simulink model "snap_poco"  (R2013a)
settings: Solver=VariableStepDiscrete  SolverMode=SingleTasking  StartTime=0.0  StopTime=4096 * 16  RelTol=1e-3
undefined symbols (not defined in the file): pfb_coeff_gen_calc
libraries: xbsIndex_r4 x15564, xps_library x54, casper_library_misc x53, xbsReplacements_r4 x42, casper_library_delays x14, simulink x1
(part 31 of 142)

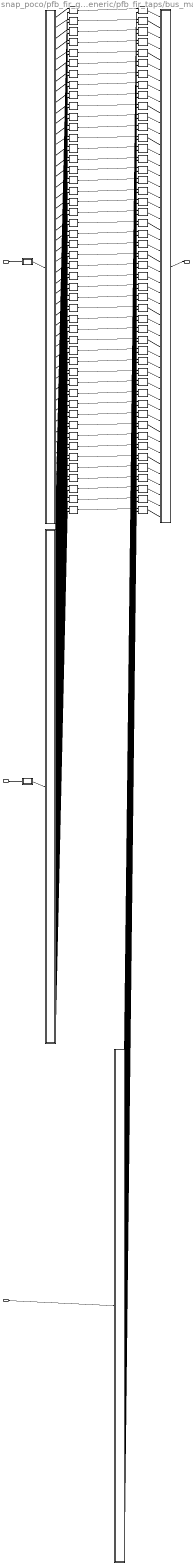
== system snap_poco/pfb_fir_generic/pfb_fir_taps/bus_madd ==
  a : Inport
  b : Inport  Port=2
  c : Inport  Port=3
  a*b+c_bussify : Subsystem  AncestorBlock=casper_library_flow_control/bus_create  mask(bus_create){inputNum=48}
      mask prompts: inputNum "Number of inputs:"
      mask init:
      | bus_create_init(gcb,...
      |     'inputNum', inputNum);
  a_debus : Subsystem  AncestorBlock=casper_library_flow_control/bus_expand  mask(bus_expand){mode=divisions of arbitrary size, outputNum=1, outputWidth=[8 8 8 8 8 8 8 8 8 8 8 8 8 8 8 8 8 8 8 8 8 8 8 8 8 8 8 8 8 8 8 8 8 8 8 8 8 8 8 8 8 8 8 8 8 8 8 8], outputBinaryPt=[7 7 7 7 7 7 7 7 7 7 7 7 7 7 7 7 7 7 7 7 7 7 7 7 7 7 7 7 7 7 7 7 7 7 7 7 7 7 7 7 7 7 7 7 7 7 7 7], outputArithmeticType=[1 1 1 1 1 1 1 1 1 1 1 1 1 1 1 1 1 1 1 1 1 1 1 1 1 1 1 1 1 1 1 1 1 1 1 1 1 1 1 1 1 1 1 1 1 1 1 1], show_format=on, outputToWorkspace=off, variablePrefix=, outputToModelAsWell=on}
      mask prompts: outputNum "Number of outputs:"; outputWidth "Output width [msb ... lsb]:"; outputBinaryPt "Output binary point position [msb ... lsb]:"; outputArithmeticType "Output arithmetic type (ufix=0, fix=1, bool=2) [msb ... lsb]:"; show_format "Print format string?"; outputToWorkspace "Output to workspace?"; variablePrefix "Variable name prefix:"; outputToModelAsWell "Output to model as well?"
      mask help:
      | Expands a 'bus' made using a bus_create or Xilinx
      | concat block.
      | The input will be divided into the specified number
      | of outputs with the specified arithmetic types.
      | Divisions are made from most significant bit.
      mask init: same as snap_poco/fft_biplex_real_2x/even_pol_debus
      settings: AttributesFormatString=48 outputs: f8.7,f8.7,f8.7,f8.7,f8.7,f8.7,f8.7,f8.7,f8.7,f8.7,f8.7,f8.7,f8.7,f8.7,f8.7,f8.7,f8.7,f8.7,f8.7,f8.7,f8.7,f8.7,f8.7,f8.7,f8.7,f8.7,f8.7,f8.7,f8.7,f8.7,f8.7,f8.7,f8.7,f8.7,f8.7,f8.7,f8.7,f8.7,f8.7,f8.7,f8.7,f8.7,f8.7,f8.7,f8.7,f8.7,f8.7,f8.7,
      mask TypeOptions mode: divisions of equal size | divisions of arbitrary size
      mask Callback mode: bus_expand_callback();
      mask Callback outputWidth: bus_expand_callback();
      mask Callback outputToWorkspace: bus_expand_callback();
  addsub{1..12} (12 alike) : xbsIndex_r4/AddSub  mode=Addition  use_carryin=off  use_carryout=off  en=off  latency=2  precision=User Defined  arith_type="Signed  (2's comp)"  n_bits=26  bin_pt=24  quantization=Truncate  overflow=Wrap  use_behavioral_HDL=on  hw_selection=Fabric  pipelined=on  dbl_ovrd=off  block_type=addsub
  addsub{13..24} (12 alike) : xbsIndex_r4/AddSub  mode=Addition  use_carryin=off  use_carryout=off  en=off  latency=2  precision=User Defined  arith_type="Signed  (2's comp)"  n_bits=27  bin_pt=24  quantization=Truncate  overflow=Wrap  use_behavioral_HDL=on  hw_selection=Fabric  pipelined=on  dbl_ovrd=off  block_type=addsub
  addsub{25..36} (12 alike) : xbsIndex_r4/AddSub  mode=Addition  use_carryin=off  use_carryout=off  en=off  latency=2  precision=User Defined  arith_type="Signed  (2's comp)"  n_bits=28  bin_pt=24  quantization=Truncate  overflow=Wrap  use_behavioral_HDL=on  hw_selection=Fabric  pipelined=on  dbl_ovrd=off  block_type=addsub
  addsub{37..48} (12 alike) : xbsIndex_r4/AddSub  mode=Addition  use_carryin=off  use_carryout=off  en=off  latency=2  precision=User Defined  arith_type="Signed  (2's comp)"  n_bits=29  bin_pt=24  quantization=Truncate  overflow=Wrap  use_behavioral_HDL=on  hw_selection=Fabric  pipelined=on  dbl_ovrd=off  block_type=addsub
  b_debus : Subsystem  AncestorBlock=casper_library_flow_control/bus_expand  mask(bus_expand){mode=divisions of arbitrary size, outputNum=1, outputWidth=[18 18 18 18 18 18 18 18 18 18 18 18 18 18 18 18 18 18 18 18 18 18 18 18 18 18 18 18 18 18 18 18 18 18 18 18 18 18 18 18 18 18 18 18 18 18 18 18], outputBinaryPt=[17 17 17 17 17 17 17 17 17 17 17 17 17 17 17 17 17 17 17 17 17 17 17 17 17 17 17 17 17 17 17 17 17 17 17 17 17 17 17 17 17 17 17 17 17 17 17 17], outputArithmeticType=[1 1 1 1 1 1 1 1 1 1 1 1 1 1 1 1 1 1 1 1 1 1 1 1 1 1 1 1 1 1 1 1 1 1 1 1 1 1 1 1 1 1 1 1 1 1 1 1], show_format=on, outputToWorkspace=off, variablePrefix=, outputToModelAsWell=on}
      mask prompts: outputNum "Number of outputs:"; outputWidth "Output width [msb ... lsb]:"; outputBinaryPt "Output binary point position [msb ... lsb]:"; outputArithmeticType "Output arithmetic type (ufix=0, fix=1, bool=2) [msb ... lsb]:"; show_format "Print format string?"; outputToWorkspace "Output to workspace?"; variablePrefix "Variable name prefix:"; outputToModelAsWell "Output to model as well?"
      mask help:
      | Expands a 'bus' made using a bus_create or Xilinx
      | concat block.
      | The input will be divided into the specified number
      | of outputs with the specified arithmetic types.
      | Divisions are made from most significant bit.
      mask init: same as snap_poco/fft_biplex_real_2x/even_pol_debus
      settings: AttributesFormatString=48 outputs: f18.17,f18.17,f18.17,f18.17,f18.17,f18.17,f18.17,f18.17,f18.17,f18.17,f18.17,f18.17,f18.17,f18.17,f18.17,f18.17,f18.17,f18.17,f18.17,f18.17,f18.17,f18.17,f18.17,f18.17,f18.17,f18.17,f18.17,f18.17,f18.17,f18.17,f18.17,f18.17,f18.17,f18.17,f18.17,f18.17,f18.17,f18.17,f18.17,f18.17,f18.17,f18.17,f18.17,f18.17,f18.17,f18.17,f18.17,f18.17,
      mask TypeOptions mode: divisions of equal size | divisions of arbitrary size
      mask Callback mode: bus_expand_callback();
      mask Callback outputWidth: bus_expand_callback();
      mask Callback outputToWorkspace: bus_expand_callback();
  c_debus : Subsystem  AncestorBlock=casper_library_flow_control/bus_expand  mask(bus_expand){mode=divisions of arbitrary size, outputNum=1, outputWidth=[26 26 26 26 26 26 26 26 26 26 26 26 26 26 26 26 26 26 26 26 26 26 26 26 27 27 27 27 27 27 27 27 27 27 27 27 28 28 28 28 28 28 28 28 28 28 28 28], outputBinaryPt=[24 24 24 24 24 24 24 24 24 24 24 24 24 24 24 24 24 24 24 24 24 24 24 24 24 24 24 24 24 24 24 24 24 24 24 24 24 24 24 24 24 24 24 24 24 24 24 24], outputArithmeticType=[1 1 1 1 1 1 1 1 1 1 1 1 1 1 1 1 1 1 1 1 1 1 1 1 1 1 1 1 1 1 1 1 1 1 1 1 1 1 1 1 1 1 1 1 1 1 1 1], show_format=on, outputToWorkspace=off, variablePrefix=, outputToModelAsWell=on}
      mask prompts: outputNum "Number of outputs:"; outputWidth "Output width [msb ... lsb]:"; outputBinaryPt "Output binary point position [msb ... lsb]:"; outputArithmeticType "Output arithmetic type (ufix=0, fix=1, bool=2) [msb ... lsb]:"; show_format "Print format string?"; outputToWorkspace "Output to workspace?"; variablePrefix "Variable name prefix:"; outputToModelAsWell "Output to model as well?"
      mask help:
      | Expands a 'bus' made using a bus_create or Xilinx
      | concat block.
      | The input will be divided into the specified number
      | of outputs with the specified arithmetic types.
      | Divisions are made from most significant bit.
      mask init: same as snap_poco/fft_biplex_real_2x/even_pol_debus
      settings: AttributesFormatString=48 outputs: f26.24,f26.24,f26.24,f26.24,f26.24,f26.24,f26.24,f26.24,f26.24,f26.24,f26.24,f26.24,f26.24,f26.24,f26.24,f26.24,f26.24,f26.24,f26.24,f26.24,f26.24,f26.24,f26.24,f26.24,f27.24,f27.24,f27.24,f27.24,f27.24,f27.24,f27.24,f27.24,f27.24,f27.24,f27.24,f27.24,f28.24,f28.24,f28.24,f28.24,f28.24,f28.24,f28.24,f28.24,f28.24,f28.24,f28.24,f28.24,
      mask TypeOptions mode: divisions of equal size | divisions of arbitrary size
      mask Callback mode: bus_expand_callback();
      mask Callback outputWidth: bus_expand_callback();
      mask Callback outputToWorkspace: bus_expand_callback();
  mult{1..48} (48 alike) : xbsIndex_r4/Mult  precision=Full  arith_type="Signed  (2's comp)"  n_bits=16  bin_pt=14  quantization=Truncate  overflow=Wrap  en=off  latency=3  use_behavioral_HDL=on  opt=Speed  use_embedded=off  optimum_pipeline=off  pipeline=on  dbl_ovrd=off  use_rpm=on  placement_style=Triangular  block_type=mult
  repa : Subsystem  AncestorBlock=casper_library_bus/bus_replicate  mask(bus_replicate){replication=1, latency=1, misc=off, implementation=core}
      mask prompts: replication "replication factor"; misc "misc support"; implementation "delay implementation"
      mask help: Output bus formed by replicating input bus a number of times
      mask init:
      | bus_replicate_init(gcb, ...
      |     'replication', replication, ...
      |     'latency', latency, ...
      |     'implementation', implementation, ...
      |     'misc', misc);
      mask TypeOptions implementation: core | behavioral
  repb : Subsystem  AncestorBlock=casper_library_bus/bus_replicate  mask(bus_replicate){replication=1, latency=1, misc=off, implementation=core}
      mask prompts: replication "replication factor"; misc "misc support"; implementation "delay implementation"
      mask help: Output bus formed by replicating input bus a number of times
      mask init:
      | bus_replicate_init(gcb, ...
      |     'replication', replication, ...
      |     'latency', latency, ...
      |     'implementation', implementation, ...
      |     'misc', misc);
      mask TypeOptions implementation: core | behavioral
  a*b+c : Outport
  wires:
  a/1 -> repa/1(in)
  b/1 -> repb/1(in)
  repa/1(out) -> a_debus/1(bus_in)
  repb/1(out) -> b_debus/1(bus_in)
  a_debus/1(msb_out48) -> mult1/1
  b_debus/1(msb_out48) -> mult1/2
  a_debus/2(out47) -> mult2/1
  b_debus/2(out47) -> mult2/2
  a_debus/3(out46) -> mult3/1
  b_debus/3(out46) -> mult3/2
  a_debus/4(out45) -> mult4/1
  b_debus/4(out45) -> mult4/2
  a_debus/5(out44) -> mult5/1
  b_debus/5(out44) -> mult5/2
  a_debus/6(out43) -> mult6/1
  b_debus/6(out43) -> mult6/2
  a_debus/7(out42) -> mult7/1
  b_debus/7(out42) -> mult7/2
  a_debus/8(out41) -> mult8/1
  b_debus/8(out41) -> mult8/2
  a_debus/9(out40) -> mult9/1
  b_debus/9(out40) -> mult9/2
  a_debus/10(out39) -> mult10/1
  b_debus/10(out39) -> mult10/2
  a_debus/11(out38) -> mult11/1
  b_debus/11(out38) -> mult11/2
  a_debus/12(out37) -> mult12/1
  b_debus/12(out37) -> mult12/2
  a_debus/13(out36) -> mult13/1
  b_debus/13(out36) -> mult13/2
  a_debus/14(out35) -> mult14/1
  b_debus/14(out35) -> mult14/2
  a_debus/15(out34) -> mult15/1
  b_debus/15(out34) -> mult15/2
  a_debus/16(out33) -> mult16/1
  b_debus/16(out33) -> mult16/2
  a_debus/17(out32) -> mult17/1
  b_debus/17(out32) -> mult17/2
  a_debus/18(out31) -> mult18/1
  b_debus/18(out31) -> mult18/2
  a_debus/19(out30) -> mult19/1
  b_debus/19(out30) -> mult19/2
  a_debus/20(out29) -> mult20/1
  b_debus/20(out29) -> mult20/2
  a_debus/21(out28) -> mult21/1
  b_debus/21(out28) -> mult21/2
  a_debus/22(out27) -> mult22/1
  b_debus/22(out27) -> mult22/2
  a_debus/23(out26) -> mult23/1
  b_debus/23(out26) -> mult23/2
  a_debus/24(out25) -> mult24/1
  b_debus/24(out25) -> mult24/2
  a_debus/25(out24) -> mult25/1
  b_debus/25(out24) -> mult25/2
  a_debus/26(out23) -> mult26/1
  b_debus/26(out23) -> mult26/2
  a_debus/27(out22) -> mult27/1
  b_debus/27(out22) -> mult27/2
  a_debus/28(out21) -> mult28/1
  b_debus/28(out21) -> mult28/2
  a_debus/29(out20) -> mult29/1
  b_debus/29(out20) -> mult29/2
  a_debus/30(out19) -> mult30/1
  b_debus/30(out19) -> mult30/2
  a_debus/31(out18) -> mult31/1
  b_debus/31(out18) -> mult31/2
  a_debus/32(out17) -> mult32/1
  b_debus/32(out17) -> mult32/2
  a_debus/33(out16) -> mult33/1
  b_debus/33(out16) -> mult33/2
  a_debus/34(out15) -> mult34/1
  b_debus/34(out15) -> mult34/2
  a_debus/35(out14) -> mult35/1
  b_debus/35(out14) -> mult35/2
  a_debus/36(out13) -> mult36/1
  b_debus/36(out13) -> mult36/2
  a_debus/37(out12) -> mult37/1
  b_debus/37(out12) -> mult37/2
  a_debus/38(out11) -> mult38/1
  b_debus/38(out11) -> mult38/2
  a_debus/39(out10) -> mult39/1
  b_debus/39(out10) -> mult39/2
  a_debus/40(out9) -> mult40/1
  b_debus/40(out9) -> mult40/2
  a_debus/41(out8) -> mult41/1
  b_debus/41(out8) -> mult41/2
  a_debus/42(out7) -> mult42/1
  b_debus/42(out7) -> mult42/2
  a_debus/43(out6) -> mult43/1
  b_debus/43(out6) -> mult43/2
  a_debus/44(out5) -> mult44/1
  b_debus/44(out5) -> mult44/2
  a_debus/45(out4) -> mult45/1
  b_debus/45(out4) -> mult45/2
  a_debus/46(out3) -> mult46/1
  b_debus/46(out3) -> mult46/2
  a_debus/47(out2) -> mult47/1
  b_debus/47(out2) -> mult47/2
  a_debus/48(lsb_out1) -> mult48/1
  b_debus/48(lsb_out1) -> mult48/2
  c/1 -> c_debus/1(bus_in)
  mult1/1 -> addsub1/1
  c_debus/1(msb_out48) -> addsub1/2
  mult2/1 -> addsub2/1
  c_debus/2(out47) -> addsub2/2
  mult3/1 -> addsub3/1
  c_debus/3(out46) -> addsub3/2
  mult4/1 -> addsub4/1
  c_debus/4(out45) -> addsub4/2
  mult5/1 -> addsub5/1
  c_debus/5(out44) -> addsub5/2
  mult6/1 -> addsub6/1
  c_debus/6(out43) -> addsub6/2
  mult7/1 -> addsub7/1
  c_debus/7(out42) -> addsub7/2
  mult8/1 -> addsub8/1
  c_debus/8(out41) -> addsub8/2
  mult9/1 -> addsub9/1
  c_debus/9(out40) -> addsub9/2
  mult10/1 -> addsub10/1
  c_debus/10(out39) -> addsub10/2
  mult11/1 -> addsub11/1
  c_debus/11(out38) -> addsub11/2
  mult12/1 -> addsub12/1
  c_debus/12(out37) -> addsub12/2
  mult13/1 -> addsub13/1
  c_debus/13(out36) -> addsub13/2
  mult14/1 -> addsub14/1
  c_debus/14(out35) -> addsub14/2
  mult15/1 -> addsub15/1
  c_debus/15(out34) -> addsub15/2
  mult16/1 -> addsub16/1
  c_debus/16(out33) -> addsub16/2
  mult17/1 -> addsub17/1
  c_debus/17(out32) -> addsub17/2
  mult18/1 -> addsub18/1
  c_debus/18(out31) -> addsub18/2
  mult19/1 -> addsub19/1
  c_debus/19(out30) -> addsub19/2
  mult20/1 -> addsub20/1
  c_debus/20(out29) -> addsub20/2
  mult21/1 -> addsub21/1
  c_debus/21(out28) -> addsub21/2
  mult22/1 -> addsub22/1
  c_debus/22(out27) -> addsub22/2
  mult23/1 -> addsub23/1
  c_debus/23(out26) -> addsub23/2
  mult24/1 -> addsub24/1
  c_debus/24(out25) -> addsub24/2
  mult25/1 -> addsub25/1
  c_debus/25(out24) -> addsub25/2
  mult26/1 -> addsub26/1
  c_debus/26(out23) -> addsub26/2
  mult27/1 -> addsub27/1
  c_debus/27(out22) -> addsub27/2
  mult28/1 -> addsub28/1
  c_debus/28(out21) -> addsub28/2
  mult29/1 -> addsub29/1
  c_debus/29(out20) -> addsub29/2
  mult30/1 -> addsub30/1
  c_debus/30(out19) -> addsub30/2
  mult31/1 -> addsub31/1
  c_debus/31(out18) -> addsub31/2
  mult32/1 -> addsub32/1
  c_debus/32(out17) -> addsub32/2
  mult33/1 -> addsub33/1
  c_debus/33(out16) -> addsub33/2
  mult34/1 -> addsub34/1
  c_debus/34(out15) -> addsub34/2
  mult35/1 -> addsub35/1
  c_debus/35(out14) -> addsub35/2
  mult36/1 -> addsub36/1
  c_debus/36(out13) -> addsub36/2
  mult37/1 -> addsub37/1
  c_debus/37(out12) -> addsub37/2
  mult38/1 -> addsub38/1
  c_debus/38(out11) -> addsub38/2
  mult39/1 -> addsub39/1
  c_debus/39(out10) -> addsub39/2
  mult40/1 -> addsub40/1
  c_debus/40(out9) -> addsub40/2
  mult41/1 -> addsub41/1
  c_debus/41(out8) -> addsub41/2
  mult42/1 -> addsub42/1
  c_debus/42(out7) -> addsub42/2
  mult43/1 -> addsub43/1
  c_debus/43(out6) -> addsub43/2
  mult44/1 -> addsub44/1
  c_debus/44(out5) -> addsub44/2
  mult45/1 -> addsub45/1
  c_debus/45(out4) -> addsub45/2
  mult46/1 -> addsub46/1
  c_debus/46(out3) -> addsub46/2
  mult47/1 -> addsub47/1
  c_debus/47(out2) -> addsub47/2
  mult48/1 -> addsub48/1
  c_debus/48(lsb_out1) -> addsub48/2
  addsub1/1 -> a*b+c_bussify/1(in1)
  addsub2/1 -> a*b+c_bussify/2(in2)
  addsub3/1 -> a*b+c_bussify/3(in3)
  addsub4/1 -> a*b+c_bussify/4(in4)
  addsub5/1 -> a*b+c_bussify/5(in5)
  addsub6/1 -> a*b+c_bussify/6(in6)
  addsub7/1 -> a*b+c_bussify/7(in7)
  addsub8/1 -> a*b+c_bussify/8(in8)
  addsub9/1 -> a*b+c_bussify/9(in9)
  addsub10/1 -> a*b+c_bussify/10(in10)
  addsub11/1 -> a*b+c_bussify/11(in11)
  addsub12/1 -> a*b+c_bussify/12(in12)
  addsub13/1 -> a*b+c_bussify/13(in13)
  addsub14/1 -> a*b+c_bussify/14(in14)
  addsub15/1 -> a*b+c_bussify/15(in15)
  addsub16/1 -> a*b+c_bussify/16(in16)
  addsub17/1 -> a*b+c_bussify/17(in17)
  addsub18/1 -> a*b+c_bussify/18(in18)
  addsub19/1 -> a*b+c_bussify/19(in19)
  addsub20/1 -> a*b+c_bussify/20(in20)
  addsub21/1 -> a*b+c_bussify/21(in21)
  addsub22/1 -> a*b+c_bussify/22(in22)
  addsub23/1 -> a*b+c_bussify/23(in23)
  addsub24/1 -> a*b+c_bussify/24(in24)
  addsub25/1 -> a*b+c_bussify/25(in25)
  addsub26/1 -> a*b+c_bussify/26(in26)
  addsub27/1 -> a*b+c_bussify/27(in27)
  addsub28/1 -> a*b+c_bussify/28(in28)
  addsub29/1 -> a*b+c_bussify/29(in29)
  addsub30/1 -> a*b+c_bussify/30(in30)
  addsub31/1 -> a*b+c_bussify/31(in31)
  addsub32/1 -> a*b+c_bussify/32(in32)
  addsub33/1 -> a*b+c_bussify/33(in33)
  addsub34/1 -> a*b+c_bussify/34(in34)
  addsub35/1 -> a*b+c_bussify/35(in35)
  addsub36/1 -> a*b+c_bussify/36(in36)
  addsub37/1 -> a*b+c_bussify/37(in37)
  addsub38/1 -> a*b+c_bussify/38(in38)
  addsub39/1 -> a*b+c_bussify/39(in39)
  addsub40/1 -> a*b+c_bussify/40(in40)
  addsub41/1 -> a*b+c_bussify/41(in41)
  addsub42/1 -> a*b+c_bussify/42(in42)
  addsub43/1 -> a*b+c_bussify/43(in43)
  addsub44/1 -> a*b+c_bussify/44(in44)
  addsub45/1 -> a*b+c_bussify/45(in45)
  addsub46/1 -> a*b+c_bussify/46(in46)
  addsub47/1 -> a*b+c_bussify/47(in47)
  addsub48/1 -> a*b+c_bussify/48(in48)
  a*b+c_bussify/1(bus_out) -> a*b+c/1

== system snap_poco/pfb_fir_generic/pfb_fir_taps/ddata0 ==
  din : Inport
  del{1..24} (24 alike) : xbsIndex_r4/Delay  rst=off  infoeditControl=Selection of Reset will increase slice count due to use of real FFs and instead of SRLs  en=off  latency=2  reg_retiming=on  dbl_ovrd=off  block_type=delay
  din_expand : Subsystem  AncestorBlock=casper_library_flow_control/bus_expand  mask(bus_expand){mode=divisions of arbitrary size, outputNum=1, outputWidth=[8  8  8  8  8  8  8  8  8  8  8  8  8  8  8  8  8  8  8  8  8  8  8  8], outputBinaryPt=[0  0  0  0  0  0  0  0  0  0  0  0  0  0  0  0  0  0  0  0  0  0  0  0], outputArithmeticType=[0  0  0  0  0  0  0  0  0  0  0  0  0  0  0  0  0  0  0  0  0  0  0  0], show_format=on, outputToWorkspace=off, variablePrefix=, outputToModelAsWell=on}
      mask prompts: outputNum "Number of outputs:"; outputWidth "Output width [msb ... lsb]:"; outputBinaryPt "Output binary point position [msb ... lsb]:"; outputArithmeticType "Output arithmetic type (ufix=0, fix=1, bool=2) [msb ... lsb]:"; show_format "Print format string?"; outputToWorkspace "Output to workspace?"; variablePrefix "Variable name prefix:"; outputToModelAsWell "Output to model as well?"
      mask help:
      | Expands a 'bus' made using a bus_create or Xilinx
      | concat block.
      | The input will be divided into the specified number
      | of outputs with the specified arithmetic types.
      | Divisions are made from most significant bit.
      mask init: same as snap_poco/fft_biplex_real_2x/even_pol_debus
      settings: AttributesFormatString=24 outputs: uf8.0,uf8.0,uf8.0,uf8.0,uf8.0,uf8.0,uf8.0,uf8.0,uf8.0,uf8.0,uf8.0,uf8.0,uf8.0,uf8.0,uf8.0,uf8.0,uf8.0,uf8.0,uf8.0,uf8.0,uf8.0,uf8.0,uf8.0,uf8.0,
      mask TypeOptions mode: divisions of equal size | divisions of arbitrary size
      mask Callback mode: bus_expand_callback();
      mask Callback outputWidth: bus_expand_callback();
      mask Callback outputToWorkspace: bus_expand_callback();
  dout_compress : Subsystem  AncestorBlock=casper_library_flow_control/bus_create  mask(bus_create){inputNum=24}
      mask prompts: inputNum "Number of inputs:"
      mask init:
      | bus_create_init(gcb,...
      |     'inputNum', inputNum);
  dout : Outport
  wires:
  din/1 -> din_expand/1(bus_in)
  din_expand/1(msb_out24) -> del1/1
  din_expand/2(out23) -> del2/1
  din_expand/3(out22) -> del3/1
  din_expand/4(out21) -> del4/1
  din_expand/5(out20) -> del5/1
  din_expand/6(out19) -> del6/1
  din_expand/7(out18) -> del7/1
  din_expand/8(out17) -> del8/1
  din_expand/9(out16) -> del9/1
  din_expand/10(out15) -> del10/1
  din_expand/11(out14) -> del11/1
  din_expand/12(out13) -> del12/1
  din_expand/13(out12) -> del13/1
  din_expand/14(out11) -> del14/1
  din_expand/15(out10) -> del15/1
  din_expand/16(out9) -> del16/1
  din_expand/17(out8) -> del17/1
  din_expand/18(out7) -> del18/1
  din_expand/19(out6) -> del19/1
  din_expand/20(out5) -> del20/1
  din_expand/21(out4) -> del21/1
  din_expand/22(out3) -> del22/1
  din_expand/23(out2) -> del23/1
  din_expand/24(lsb_out1) -> del24/1
  del1/1 -> dout_compress/1(in1)
  del2/1 -> dout_compress/2(in2)
  del3/1 -> dout_compress/3(in3)
  del4/1 -> dout_compress/4(in4)
  del5/1 -> dout_compress/5(in5)
  del6/1 -> dout_compress/6(in6)
  del7/1 -> dout_compress/7(in7)
  del8/1 -> dout_compress/8(in8)
  del9/1 -> dout_compress/9(in9)
  del10/1 -> dout_compress/10(in10)
  del11/1 -> dout_compress/11(in11)
  del12/1 -> dout_compress/12(in12)
  del13/1 -> dout_compress/13(in13)
  del14/1 -> dout_compress/14(in14)
  del15/1 -> dout_compress/15(in15)
  del16/1 -> dout_compress/16(in16)
  del17/1 -> dout_compress/17(in17)
  del18/1 -> dout_compress/18(in18)
  del19/1 -> dout_compress/19(in19)
  del20/1 -> dout_compress/20(in20)
  del21/1 -> dout_compress/21(in21)
  del22/1 -> dout_compress/22(in22)
  del23/1 -> dout_compress/23(in23)
  del24/1 -> dout_compress/24(in24)
  dout_compress/1(bus_out) -> dout/1

== system snap_poco/pfb_fir_generic/pfb_fir_taps/ddata1 ==
  din : Inport
  del{1..36} (36 alike) : xbsIndex_r4/Delay  rst=off  infoeditControl=Selection of Reset will increase slice count due to use of real FFs and instead of SRLs  en=off  latency=2  reg_retiming=on  dbl_ovrd=off  block_type=delay
  din_expand : Subsystem  AncestorBlock=casper_library_flow_control/bus_expand  mask(bus_expand){mode=divisions of arbitrary size, outputNum=1, outputWidth=[8  8  8  8  8  8  8  8  8  8  8  8  8  8  8  8  8  8  8  8  8  8  8  8  8  8  8  8  8  8  8  8  8  8  8  8], outputBinaryPt=[0  0  0  0  0  0  0  0  0  0  0  0  0  0  0  0  0  0  0  0  0  0  0  0  0  0  0  0  0  0  0  0  0  0  0  0], outputArithmeticType=[0  0  0  0  0  0  0  0  0  0  0  0  0  0  0  0  0  0  0  0  0  0  0  0  0  0  0  0  0  0  0  0  0  0  0  0], show_format=on, outputToWorkspace=off, variablePrefix=, outputToModelAsWell=on}
      mask prompts: outputNum "Number of outputs:"; outputWidth "Output width [msb ... lsb]:"; outputBinaryPt "Output binary point position [msb ... lsb]:"; outputArithmeticType "Output arithmetic type (ufix=0, fix=1, bool=2) [msb ... lsb]:"; show_format "Print format string?"; outputToWorkspace "Output to workspace?"; variablePrefix "Variable name prefix:"; outputToModelAsWell "Output to model as well?"
      mask help:
      | Expands a 'bus' made using a bus_create or Xilinx
      | concat block.
      | The input will be divided into the specified number
      | of outputs with the specified arithmetic types.
      | Divisions are made from most significant bit.
      mask init: same as snap_poco/fft_biplex_real_2x/even_pol_debus
      settings: AttributesFormatString=36 outputs: uf8.0,uf8.0,uf8.0,uf8.0,uf8.0,uf8.0,uf8.0,uf8.0,uf8.0,uf8.0,uf8.0,uf8.0,uf8.0,uf8.0,uf8.0,uf8.0,uf8.0,uf8.0,uf8.0,uf8.0,uf8.0,uf8.0,uf8.0,uf8.0,uf8.0,uf8.0,uf8.0,uf8.0,uf8.0,uf8.0,uf8.0,uf8.0,uf8.0,uf8.0,uf8.0,uf8.0,
      mask TypeOptions mode: divisions of equal size | divisions of arbitrary size
      mask Callback mode: bus_expand_callback();
      mask Callback outputWidth: bus_expand_callback();
      mask Callback outputToWorkspace: bus_expand_callback();
  dout_compress : Subsystem  AncestorBlock=casper_library_flow_control/bus_create  mask(bus_create){inputNum=36}
      mask prompts: inputNum "Number of inputs:"
      mask init:
      | bus_create_init(gcb,...
      |     'inputNum', inputNum);
  dout : Outport
  wires:
  din/1 -> din_expand/1(bus_in)
  din_expand/1(msb_out36) -> del1/1
  din_expand/2(out35) -> del2/1
  din_expand/3(out34) -> del3/1
  din_expand/4(out33) -> del4/1
  din_expand/5(out32) -> del5/1
  din_expand/6(out31) -> del6/1
  din_expand/7(out30) -> del7/1
  din_expand/8(out29) -> del8/1
  din_expand/9(out28) -> del9/1
  din_expand/10(out27) -> del10/1
  din_expand/11(out26) -> del11/1
  din_expand/12(out25) -> del12/1
  din_expand/13(out24) -> del13/1
  din_expand/14(out23) -> del14/1
  din_expand/15(out22) -> del15/1
  din_expand/16(out21) -> del16/1
  din_expand/17(out20) -> del17/1
  din_expand/18(out19) -> del18/1
  din_expand/19(out18) -> del19/1
  din_expand/20(out17) -> del20/1
  din_expand/21(out16) -> del21/1
  din_expand/22(out15) -> del22/1
  din_expand/23(out14) -> del23/1
  din_expand/24(out13) -> del24/1
  din_expand/25(out12) -> del25/1
  din_expand/26(out11) -> del26/1
  din_expand/27(out10) -> del27/1
  din_expand/28(out9) -> del28/1
  din_expand/29(out8) -> del29/1
  din_expand/30(out7) -> del30/1
  din_expand/31(out6) -> del31/1
  din_expand/32(out5) -> del32/1
  din_expand/33(out4) -> del33/1
  din_expand/34(out3) -> del34/1
  din_expand/35(out2) -> del35/1
  din_expand/36(lsb_out1) -> del36/1
  del1/1 -> dout_compress/1(in1)
  del2/1 -> dout_compress/2(in2)
  del3/1 -> dout_compress/3(in3)
  del4/1 -> dout_compress/4(in4)
  del5/1 -> dout_compress/5(in5)
  del6/1 -> dout_compress/6(in6)
  del7/1 -> dout_compress/7(in7)
  del8/1 -> dout_compress/8(in8)
  del9/1 -> dout_compress/9(in9)
  del10/1 -> dout_compress/10(in10)
  del11/1 -> dout_compress/11(in11)
  del12/1 -> dout_compress/12(in12)
  del13/1 -> dout_compress/13(in13)
  del14/1 -> dout_compress/14(in14)
  del15/1 -> dout_compress/15(in15)
  del16/1 -> dout_compress/16(in16)
  del17/1 -> dout_compress/17(in17)
  del18/1 -> dout_compress/18(in18)
  del19/1 -> dout_compress/19(in19)
  del20/1 -> dout_compress/20(in20)
  del21/1 -> dout_compress/21(in21)
  del22/1 -> dout_compress/22(in22)
  del23/1 -> dout_compress/23(in23)
  del24/1 -> dout_compress/24(in24)
  del25/1 -> dout_compress/25(in25)
  del26/1 -> dout_compress/26(in26)
  del27/1 -> dout_compress/27(in27)
  del28/1 -> dout_compress/28(in28)
  del29/1 -> dout_compress/29(in29)
  del30/1 -> dout_compress/30(in30)
  del31/1 -> dout_compress/31(in31)
  del32/1 -> dout_compress/32(in32)
  del33/1 -> dout_compress/33(in33)
  del34/1 -> dout_compress/34(in34)
  del35/1 -> dout_compress/35(in35)
  del36/1 -> dout_compress/36(in36)
  dout_compress/1(bus_out) -> dout/1

== system snap_poco/pfb_fir_generic/pfb_fir_taps/delay_bram ==
  addr : Inport
  din : Inport  Port=2
  we : Inport  Port=3
  bram{0..31} (32 alike) : xbsIndex_r4/Single Port RAM  depth=2048  initVector=getfield(get_param(gcb, 'UserData'), 'initVector')  distributed_mem=Block RAM  write_mode=Read Before Write  rst=off  init_reg=0  en=off  latency=1  optimize=Area  dbl_ovrd=off  block_type=spram
  ddin : xbsIndex_r4/Delay  rst=off  infoeditControl=Selection of Reset will increase slice count due to use of real FFs and instead of SRLs  en=off  latency=0  reg_retiming=on  dbl_ovrd=off  block_type=delay
  debus_addr : Subsystem  AncestorBlock=casper_library_flow_control/bus_expand  mask(bus_expand){mode=divisions of equal size, outputNum=32, outputWidth=[11 11 11 11 11 11 11 11 11 11 11 11 11 11 11 11 11 11 11 11 11 11 11 11 11 11 11 11 11 11 11 11], outputBinaryPt=[0 0 0 0 0 0 0 0 0 0 0 0 0 0 0 0 0 0 0 0 0 0 0 0 0 0 0 0 0 0 0 0], outputArithmeticType=[0 0 0 0 0 0 0 0 0 0 0 0 0 0 0 0 0 0 0 0 0 0 0 0 0 0 0 0 0 0 0 0], show_format=on, outputToWorkspace=off, variablePrefix=, outputToModelAsWell=on}
      mask prompts: outputNum "Number of outputs:"; outputWidth "Output width:"; outputBinaryPt "Output binary point position:"; outputArithmeticType "Output arithmetic type (ufix=0, fix=1, bool=2):"; show_format "Print format string?"; outputToWorkspace "Output to workspace?"; variablePrefix "Variable name prefix:"; outputToModelAsWell "Output to model as well?"
      mask help:
      | Expands a 'bus' made using a bus_create or Xilinx
      | concat block.
      | The input will be divided into the specified number
      | of outputs with the specified arithmetic types.
      | Divisions are made from most significant bit.
      mask init: same as snap_poco/fft_biplex_real_2x/even_pol_debus
      settings: AttributesFormatString=32 outputs: uf11.0,uf11.0,uf11.0,uf11.0,uf11.0,uf11.0,uf11.0,uf11.0,uf11.0,uf11.0,uf11.0,uf11.0,uf11.0,uf11.0,uf11.0,uf11.0,uf11.0,uf11.0,uf11.0,uf11.0,uf11.0,uf11.0,uf11.0,uf11.0,uf11.0,uf11.0,uf11.0,uf11.0,uf11.0,uf11.0,uf11.0,uf11.0,
      mask TypeOptions mode: divisions of equal size | divisions of arbitrary size
      mask Callback mode: bus_expand_callback();
      mask Callback outputWidth: bus_expand_callback();
      mask Callback outputToWorkspace: bus_expand_callback();
  debus_din : Subsystem  AncestorBlock=casper_library_flow_control/bus_expand  mask(bus_expand){mode=divisions of arbitrary size, outputNum=1, outputWidth=[9 9 9 9 9 9 9 9 9 9 9 9 9 9 9 9 9 9 9 9 9 9 9 9 9 9 9 9 9 9 9 9], outputBinaryPt=[0 0 0 0 0 0 0 0 0 0 0 0 0 0 0 0 0 0 0 0 0 0 0 0 0 0 0 0 0 0 0 0], outputArithmeticType=[0 0 0 0 0 0 0 0 0 0 0 0 0 0 0 0 0 0 0 0 0 0 0 0 0 0 0 0 0 0 0 0], show_format=on, outputToWorkspace=off, variablePrefix=, outputToModelAsWell=on}
      mask prompts: outputNum "Number of outputs:"; outputWidth "Output width [msb ... lsb]:"; outputBinaryPt "Output binary point position [msb ... lsb]:"; outputArithmeticType "Output arithmetic type (ufix=0, fix=1, bool=2) [msb ... lsb]:"; show_format "Print format string?"; outputToWorkspace "Output to workspace?"; variablePrefix "Variable name prefix:"; outputToModelAsWell "Output to model as well?"
      mask help:
      | Expands a 'bus' made using a bus_create or Xilinx
      | concat block.
      | The input will be divided into the specified number
      | of outputs with the specified arithmetic types.
      | Divisions are made from most significant bit.
      mask init: same as snap_poco/fft_biplex_real_2x/even_pol_debus
      settings: AttributesFormatString=32 outputs: uf9.0,uf9.0,uf9.0,uf9.0,uf9.0,uf9.0,uf9.0,uf9.0,uf9.0,uf9.0,uf9.0,uf9.0,uf9.0,uf9.0,uf9.0,uf9.0,uf9.0,uf9.0,uf9.0,uf9.0,uf9.0,uf9.0,uf9.0,uf9.0,uf9.0,uf9.0,uf9.0,uf9.0,uf9.0,uf9.0,uf9.0,uf9.0,
      mask TypeOptions mode: divisions of equal size | divisions of arbitrary size
      mask Callback mode: bus_expand_callback();
      mask Callback outputWidth: bus_expand_callback();
      mask Callback outputToWorkspace: bus_expand_callback();
  debus_we : Subsystem  AncestorBlock=casper_library_flow_control/bus_expand  mask(bus_expand){mode=divisions of equal size, outputNum=32, outputWidth=[1 1 1 1 1 1 1 1 1 1 1 1 1 1 1 1 1 1 1 1 1 1 1 1 1 1 1 1 1 1 1 1], outputBinaryPt=[0 0 0 0 0 0 0 0 0 0 0 0 0 0 0 0 0 0 0 0 0 0 0 0 0 0 0 0 0 0 0 0], outputArithmeticType=[2 2 2 2 2 2 2 2 2 2 2 2 2 2 2 2 2 2 2 2 2 2 2 2 2 2 2 2 2 2 2 2], show_format=on, outputToWorkspace=off, variablePrefix=, outputToModelAsWell=on}
      mask prompts: outputNum "Number of outputs:"; outputWidth "Output width:"; outputBinaryPt "Output binary point position:"; outputArithmeticType "Output arithmetic type (ufix=0, fix=1, bool=2):"; show_format "Print format string?"; outputToWorkspace "Output to workspace?"; variablePrefix "Variable name prefix:"; outputToModelAsWell "Output to model as well?"
      mask help:
      | Expands a 'bus' made using a bus_create or Xilinx
      | concat block.
      | The input will be divided into the specified number
      | of outputs with the specified arithmetic types.
      | Divisions are made from most significant bit.
      mask init: same as snap_poco/fft_biplex_real_2x/even_pol_debus
      settings: AttributesFormatString=32 outputs: b,b,b,b,b,b,b,b,b,b,b,b,b,b,b,b,b,b,b,b,b,b,b,b,b,b,b,b,b,b,b,b,
      mask TypeOptions mode: divisions of equal size | divisions of arbitrary size
      mask Callback mode: bus_expand_callback();
      mask Callback outputWidth: bus_expand_callback();
      mask Callback outputToWorkspace: bus_expand_callback();
  din_bussify : Subsystem  AncestorBlock=casper_library_flow_control/bus_create  mask(bus_create){inputNum=32}
      mask prompts: inputNum "Number of inputs:"
      mask init:
      | bus_create_init(gcb,...
      |     'inputNum', inputNum);
  rep_addr : Subsystem  AncestorBlock=casper_library_bus/bus_replicate  mask(bus_replicate){replication=32, latency=1, misc=off, implementation=core}
      mask prompts: replication "replication factor"; misc "misc support"; implementation "delay implementation"
      mask help: Output bus formed by replicating input bus a number of times
      mask init:
      | bus_replicate_init(gcb, ...
      |     'replication', replication, ...
      |     'latency', latency, ...
      |     'implementation', implementation, ...
      |     'misc', misc);
      mask TypeOptions implementation: core | behavioral
  rep_we : Subsystem  AncestorBlock=casper_library_bus/bus_replicate  mask(bus_replicate){replication=32, latency=0, misc=off, implementation=behavioral}
      mask prompts: replication "replication factor"; misc "misc support"; implementation "delay implementation"
      mask help: Output bus formed by replicating input bus a number of times
      mask init:
      | bus_replicate_init(gcb, ...
      |     'replication', replication, ...
      |     'latency', latency, ...
      |     'implementation', implementation, ...
      |     'misc', misc);
      mask TypeOptions implementation: core | behavioral
  dout : Outport
  wires:
  addr/1 -> rep_addr/1(in)
  din/1 -> ddin/1
  we/1 -> rep_we/1(in)
  rep_addr/1(out) -> debus_addr/1(bus_in)
  ddin/1 -> debus_din/1(bus_in)
  rep_we/1(out) -> debus_we/1(bus_in)
  debus_addr/1(msb_out32) -> bram0/1
  debus_din/1(msb_out32) -> bram0/2
  debus_we/1(msb_out32) -> bram0/3
  debus_addr/2(out31) -> bram1/1
  debus_din/2(out31) -> bram1/2
  debus_we/2(out31) -> bram1/3
  debus_addr/3(out30) -> bram2/1
  debus_din/3(out30) -> bram2/2
  debus_we/3(out30) -> bram2/3
  debus_addr/4(out29) -> bram3/1
  debus_din/4(out29) -> bram3/2
  debus_we/4(out29) -> bram3/3
  debus_addr/5(out28) -> bram4/1
  debus_din/5(out28) -> bram4/2
  debus_we/5(out28) -> bram4/3
  debus_addr/6(out27) -> bram5/1
  debus_din/6(out27) -> bram5/2
  debus_we/6(out27) -> bram5/3
  debus_addr/7(out26) -> bram6/1
  debus_din/7(out26) -> bram6/2
  debus_we/7(out26) -> bram6/3
  debus_addr/8(out25) -> bram7/1
  debus_din/8(out25) -> bram7/2
  debus_we/8(out25) -> bram7/3
  debus_addr/9(out24) -> bram8/1
  debus_din/9(out24) -> bram8/2
  debus_we/9(out24) -> bram8/3
  debus_addr/10(out23) -> bram9/1
  debus_din/10(out23) -> bram9/2
  debus_we/10(out23) -> bram9/3
  debus_addr/11(out22) -> bram10/1
  debus_din/11(out22) -> bram10/2
  debus_we/11(out22) -> bram10/3
  debus_addr/12(out21) -> bram11/1
  debus_din/12(out21) -> bram11/2
  debus_we/12(out21) -> bram11/3
  debus_addr/13(out20) -> bram12/1
  debus_din/13(out20) -> bram12/2
  debus_we/13(out20) -> bram12/3
  debus_addr/14(out19) -> bram13/1
  debus_din/14(out19) -> bram13/2
  debus_we/14(out19) -> bram13/3
  debus_addr/15(out18) -> bram14/1
  debus_din/15(out18) -> bram14/2
  debus_we/15(out18) -> bram14/3
  debus_addr/16(out17) -> bram15/1
  debus_din/16(out17) -> bram15/2
  debus_we/16(out17) -> bram15/3
  debus_addr/17(out16) -> bram16/1
  debus_din/17(out16) -> bram16/2
  debus_we/17(out16) -> bram16/3
  debus_addr/18(out15) -> bram17/1
  debus_din/18(out15) -> bram17/2
  debus_we/18(out15) -> bram17/3
  debus_addr/19(out14) -> bram18/1
  debus_din/19(out14) -> bram18/2
  debus_we/19(out14) -> bram18/3
  debus_addr/20(out13) -> bram19/1
  debus_din/20(out13) -> bram19/2
  debus_we/20(out13) -> bram19/3
  debus_addr/21(out12) -> bram20/1
  debus_din/21(out12) -> bram20/2
  debus_we/21(out12) -> bram20/3
  debus_addr/22(out11) -> bram21/1
  debus_din/22(out11) -> bram21/2
  debus_we/22(out11) -> bram21/3
  debus_addr/23(out10) -> bram22/1
  debus_din/23(out10) -> bram22/2
  debus_we/23(out10) -> bram22/3
  debus_addr/24(out9) -> bram23/1
  debus_din/24(out9) -> bram23/2
  debus_we/24(out9) -> bram23/3
  debus_addr/25(out8) -> bram24/1
  debus_din/25(out8) -> bram24/2
  debus_we/25(out8) -> bram24/3
  debus_addr/26(out7) -> bram25/1
  debus_din/26(out7) -> bram25/2
  debus_we/26(out7) -> bram25/3
  debus_addr/27(out6) -> bram26/1
  debus_din/27(out6) -> bram26/2
  debus_we/27(out6) -> bram26/3
  debus_addr/28(out5) -> bram27/1
  debus_din/28(out5) -> bram27/2
  debus_we/28(out5) -> bram27/3
  debus_addr/29(out4) -> bram28/1
  debus_din/29(out4) -> bram28/2
  debus_we/29(out4) -> bram28/3
  debus_addr/30(out3) -> bram29/1
  debus_din/30(out3) -> bram29/2
  debus_we/30(out3) -> bram29/3
  debus_addr/31(out2) -> bram30/1
  debus_din/31(out2) -> bram30/2
  debus_we/31(out2) -> bram30/3
  debus_addr/32(lsb_out1) -> bram31/1
  debus_din/32(lsb_out1) -> bram31/2
  debus_we/32(lsb_out1) -> bram31/3
  bram0/1 -> din_bussify/1(in1)
  bram1/1 -> din_bussify/2(in2)
  bram2/1 -> din_bussify/3(in3)
  bram3/1 -> din_bussify/4(in4)
  bram4/1 -> din_bussify/5(in5)
  bram5/1 -> din_bussify/6(in6)
  bram6/1 -> din_bussify/7(in7)
  bram7/1 -> din_bussify/8(in8)
  bram8/1 -> din_bussify/9(in9)
  bram9/1 -> din_bussify/10(in10)
  bram10/1 -> din_bussify/11(in11)
  bram11/1 -> din_bussify/12(in12)
  bram12/1 -> din_bussify/13(in13)
  bram13/1 -> din_bussify/14(in14)
  bram14/1 -> din_bussify/15(in15)
  bram15/1 -> din_bussify/16(in16)
  bram16/1 -> din_bussify/17(in17)
  bram17/1 -> din_bussify/18(in18)
  bram18/1 -> din_bussify/19(in19)
  bram19/1 -> din_bussify/20(in20)
  bram20/1 -> din_bussify/21(in21)
  bram21/1 -> din_bussify/22(in22)
  bram22/1 -> din_bussify/23(in23)
  bram23/1 -> din_bussify/24(in24)
  bram24/1 -> din_bussify/25(in25)
  bram25/1 -> din_bussify/26(in26)
  bram26/1 -> din_bussify/27(in27)
  bram27/1 -> din_bussify/28(in28)
  bram28/1 -> din_bussify/29(in29)
  bram29/1 -> din_bussify/30(in30)
  bram30/1 -> din_bussify/31(in31)
  bram31/1 -> din_bussify/32(in32)
  din_bussify/1(bus_out) -> dout/1

== system snap_poco/snap_fft_in/add_gen/edge_detect ==
  in : Inport
  Delay : xbsIndex_r4/Delay  rst=off  infoeditControl=Selection of Reset will increase slice count due to use of real FFs and instead of SRLs  en=off  latency=1  reg_retiming=off  dbl_ovrd=off  block_type=delay
      settings: xl_area=[0, 0, 0, 0, 0, 0, 0]
  Inverter : xbsIndex_r4/Inverter  en=off  latency=0  dbl_ovrd=off  block_type=inv
      settings: xl_area=[0, 0, 0, 0, 0, 0, 0]
  edge_op : xbsIndex_r4/Logical  logical_function=XNOR  inputs=2  en=off  latency=0  precision=Full  arith_type=Unsigned  n_bits=8  bin_pt=2  align_bp=on  dbl_ovrd=off  block_type=logical
      settings: xl_area=[0, 0, 0, 0, 0, 0, 0]
  out : Outport
  wires:
  Delay/1 -> edge_op/2
  in/1 -> Delay/1, Inverter/1
  edge_op/1 -> out/1
  Inverter/1 -> edge_op/1

== system snap_poco/snap_fft_in/basic_ctrl/dram_munge ==
  note: Buffer 4 input words when using DRAM
      | then combine and output the first two,
      | then second. Ensures that a full burst
      | goes through every time so that status
      | register records number of bytes fully in
      | DRAM
  note: Choose DRAM data
      | or standard. Constant input
      | to muxes should ensure
      | other path optimised
      | away
  note: 1st output same time
      | as last input
  vin : Inport
  din : Inport  Port=2
  we : Inport  Port=3
  init : Inport  Port=4
  Concat : xbsIndex_r4/Concat  num_inputs=4  dbl_ovrd=off  block_type=concat
  Concat1 : xbsIndex_r4/Concat  num_inputs=4  dbl_ovrd=off  block_type=concat
  Constant : xbsIndex_r4/Constant  const=0  gui_display_data_type=Fixed-point  arith_type=Unsigned  n_bits=8  bin_pt=0  preci_type=Single  exp_width=8  frac_width=24  explicit_period=on  period=1  equ=P=C  opselect=C  inp2=PCIN>>17  opr=+  inp1=P  carry=CIN  dbl_ovrd=off  block_type=constant
      settings: block_version=11.4
  Delay : xbsIndex_r4/Delay  rst=off  infoeditControl=Selection of Reset will increase slice count due to use of real FFs and instead of SRLs  en=off  latency=1  reg_retiming=off  dbl_ovrd=off  block_type=delay
      settings: block_version=11.4
  Delay1 : xbsIndex_r4/Delay  rst=off  infoeditControl=Selection of Reset will increase slice count due to use of real FFs and instead of SRLs  en=off  latency=1  reg_retiming=off  dbl_ovrd=off  block_type=delay
      settings: block_version=11.4
  Logical : xbsIndex_r4/Logical  logical_function=AND  inputs=2  en=off  latency=1  precision=Full  arith_type=Unsigned  n_bits=16  bin_pt=0  align_bp=on  dbl_ovrd=off  block_type=logical
      settings: block_version=11.4
  Logical1 : xbsIndex_r4/Logical  logical_function=OR  inputs=2  en=off  latency=0  precision=Full  arith_type=Unsigned  n_bits=16  bin_pt=0  align_bp=on  dbl_ovrd=off  block_type=logical
      settings: block_version=11.4
  Logical2 : xbsIndex_r4/Logical  logical_function=AND  inputs=2  en=off  latency=0  precision=Full  arith_type=Unsigned  n_bits=16  bin_pt=0  align_bp=on  dbl_ovrd=off  block_type=logical
      settings: block_version=11.4
  Mux1 : xbsIndex_r4/Mux  inputs=2  en=off  latency=1  precision=Full  arith_type=Unsigned  n_bits=16  bin_pt=14  quantization=Truncate  overflow=Wrap  dbl_ovrd=off  block_type=mux
      settings: block_version=11.4
  Register{,1..3,5} (5 alike) : xbsIndex_r4/Register  init=0  rst=off  en=on  dbl_ovrd=off  block_type=register
      settings: block_version=11.4
  Register4 : xbsIndex_r4/Register  init=0  rst=on  en=on  dbl_ovrd=off  block_type=register
      settings: block_version=11.4
  Relational{,1..3} (4 alike) : xbsIndex_r4/Relational  mode=a=b  op_type=Bool  en=off  latency=0  dbl_ovrd=off  block_type=relational
  con0 : xbsIndex_r4/Constant  const=0  gui_display_data_type=Fixed-point  arith_type=Unsigned  n_bits=2  bin_pt=0  preci_type=Single  exp_width=8  frac_width=24  explicit_period=on  period=1  equ=P=C  opselect=C  inp2=PCIN>>17  opr=+  inp1=P  carry=CIN  dbl_ovrd=off  block_type=constant
      settings: block_version=11.4
  con1 : xbsIndex_r4/Constant  const=1  gui_display_data_type=Fixed-point  arith_type=Unsigned  n_bits=2  bin_pt=0  preci_type=Single  exp_width=8  frac_width=24  explicit_period=on  period=1  equ=P=C  opselect=C  inp2=PCIN>>17  opr=+  inp1=P  carry=CIN  dbl_ovrd=off  block_type=constant
      settings: block_version=11.4
  con2 : xbsIndex_r4/Constant  const=2  gui_display_data_type=Fixed-point  arith_type=Unsigned  n_bits=2  bin_pt=0  preci_type=Single  exp_width=8  frac_width=24  explicit_period=on  period=1  equ=P=C  opselect=C  inp2=PCIN>>17  opr=+  inp1=P  carry=CIN  dbl_ovrd=off  block_type=constant
      settings: block_version=11.4
  con3 : xbsIndex_r4/Constant  const=3  gui_display_data_type=Fixed-point  arith_type=Unsigned  n_bits=2  bin_pt=0  preci_type=Single  exp_width=8  frac_width=24  explicit_period=on  period=1  equ=P=C  opselect=C  inp2=PCIN>>17  opr=+  inp1=P  carry=CIN  dbl_ovrd=off  block_type=constant
      settings: block_version=11.4
  data_choice : xbsIndex_r4/Mux  inputs=2  en=off  latency=0  precision=User Defined  arith_type=Unsigned  n_bits=32  bin_pt=0  quantization=Truncate  overflow=Wrap  dbl_ovrd=off  block_type=mux
      settings: block_version=11.4
  dout_count : xbsIndex_r4/Counter  cnt_type=Free Running  cnt_to=Inf  operation=Up  start_count=0  cnt_by_val=1  arith_type=Unsigned  n_bits=1  bin_pt=0  load_pin=off  rst=on  en=on  explicit_period=on  period=1  use_behavioral_HDL=off  implementation=Fabric  dbl_ovrd=off  block_type=counter
      settings: block_version=11.4
  dram : xbsIndex_r4/Constant  const=0  gui_display_data_type=Fixed-point  arith_type=Boolean  n_bits=16  bin_pt=14  preci_type=Single  exp_width=8  frac_width=24  explicit_period=on  period=1  equ=P=C  opselect=C  inp2=PCIN>>17  opr=+  inp1=P  carry=CIN  dbl_ovrd=off  block_type=constant
      settings: block_version=11.4
  input_count : xbsIndex_r4/Counter  cnt_type=Free Running  cnt_to=Inf  operation=Up  start_count=0  cnt_by_val=1  arith_type=Unsigned  n_bits=2  bin_pt=0  load_pin=off  rst=on  en=on  explicit_period=on  period=1  use_behavioral_HDL=off  implementation=Fabric  dbl_ovrd=off  block_type=counter
      settings: block_version=11.4
  vout_choice : xbsIndex_r4/Mux  inputs=2  en=off  latency=0  precision=Full  arith_type=Unsigned  n_bits=16  bin_pt=14  quantization=Truncate  overflow=Wrap  dbl_ovrd=off  block_type=mux
      settings: block_version=11.4
  we_choice : xbsIndex_r4/Mux  inputs=2  en=off  latency=0  precision=Full  arith_type=Unsigned  n_bits=16  bin_pt=14  quantization=Truncate  overflow=Wrap  dbl_ovrd=off  block_type=mux
      settings: block_version=11.4
  vout : Outport
  dout : Outport  Port=2
  we_o : Outport  Port=3
  wires:
  data_choice/1 -> dout/1
  init/1 -> input_count/1, [init]
  we/1 -> input_count/2, Logical/2, [we]
  din/1 -> Register/1, Register1/1, Register2/1, Register3/1, [din]
  input_count/1 -> Relational/1, Relational1/1, Relational2/1, Relational3/1
  con0/1 -> Relational/2
  con1/1 -> Relational1/2
  con2/1 -> Relational2/2
  con3/1 -> Relational3/2
  Relational/1 -> Register/2
  Relational1/1 -> Register1/2
  Relational2/1 -> Register2/2
  Relational3/1 -> Register3/2, Logical/1
  Logical/1 -> Delay/1, Logical1/1
  Delay/1 -> Logical1/2
  Concat/1 -> Mux1/2
  Concat1/1 -> Mux1/3
  Logical1/1 -> dout_count/2, Delay1/1
  [init] -> dout_count/1
  dout_count/1 -> Mux1/1
  we_choice/1 -> we_o/1
  Delay1/1 -> we_choice/3
  [we] -> we_choice/2
  Mux1/1 -> data_choice/3
  [din] -> data_choice/2
  dram/1 -> data_choice/1, we_choice/1, vout_choice/1
  [init] -> Register4/1, Register4/3
  Register4/1 -> Logical2/1
  vin/1 -> Register5/1, [vin]
  [we] -> Register4/2, Logical2/2
  Logical2/1 -> Register5/2
  vout_choice/1 -> vout/1
  Register5/1 -> vout_choice/3
  [vin] -> vout_choice/2
  Register/1 -> Concat/2
  Register1/1 -> Concat/4
  Constant/1 -> Concat/1, Concat/3, Concat1/1, Concat1/3
  Register2/1 -> Concat1/2
  Register3/1 -> Concat1/4

== system snap_poco/snap_fft_out/add_gen/edge_detect ==
  in : Inport
  Delay : xbsIndex_r4/Delay  rst=off  infoeditControl=Selection of Reset will increase slice count due to use of real FFs and instead of SRLs  en=off  latency=1  reg_retiming=off  dbl_ovrd=off  block_type=delay
      settings: xl_area=[0, 0, 0, 0, 0, 0, 0]
  Inverter : xbsIndex_r4/Inverter  en=off  latency=0  dbl_ovrd=off  block_type=inv
      settings: xl_area=[0, 0, 0, 0, 0, 0, 0]
  edge_op : xbsIndex_r4/Logical  logical_function=XNOR  inputs=2  en=off  latency=0  precision=Full  arith_type=Unsigned  n_bits=8  bin_pt=2  align_bp=on  dbl_ovrd=off  block_type=logical
      settings: xl_area=[0, 0, 0, 0, 0, 0, 0]
  out : Outport
  wires:
  Inverter/1 -> edge_op/1
  edge_op/1 -> out/1
  in/1 -> Inverter/1, Delay/1
  Delay/1 -> edge_op/2
